simulink model "test storgrossenbeobachter"  (R2025b)
settings: Solver=ode23s  StartTime=0  StopTime=100  FixedStep=tStep  RelTol=1e-3  EnableMultiTasking=on
values from neighbouring files (symbols this model uses):
  A = [0 1 0 0 ... (first row only)    [test_init.m]    (also in zustandsregler.m)
  B = [0; -30.49; 0; 30.49]    [reglerInit.m]    (also in test_init.m; zustandsregler.m)
  C_new = [1 0 0 0 ... (first row only)    [reglerInit.m]    (also in test_init.m; zustandsregler.m)
  E_temp = zeros(4, 12)    [reglerInit.m]    (also in test_init.m)
  G = [1;1;1;1]    [reglerInit.m]    (also in test_init.m)
  Gamma_temp = zeros(6, 4)    [reglerInit.m]    (also in test_init.m)
  Kx = zeros(6, 4)    [reglerInit.m]    (also in test_init.m)
  Kxi = zeros(6,4)    [reglerInit.m]    (also in test_init.m)
  m1 = m1_sim    (= 1)    [test_init.m]    (also in zustandsregler.m)
  Pi_temp = zeros(4, 24)    [reglerInit.m]    (also in test_init.m)
  S_sy = [0 0 0 0 ... (first row only)    [reglerInit.m]    (also in test_init.m; zustandsregler.m)
  T = [0.3,1.2,1.5,1.7,1.7,3]    [reglerInit.m]    (also in test_init.m = [3,3,1.5,2,2.3,3]; zustandsregler.m = 50)
  x0 = [0; 0; 0; 0]    [reglerInit.m]    (also in test_init.m; zustandsregler.m = [0; 0; 1; 0])
  x_soll = 2    [test_init.m]
  xi0 = [0;0;0;0]    [reglerInit.m]    (also in test_init.m; zustandsregler.m = 0)
  zhut0 = [0;0;0;0]    [reglerInit.m]    (also in test_init.m; zustandsregler.m)
settings Model: Creator=Henning Schlüter  LastModifiedBy=marin
settings SolverCC: AlgebraicLoopSolver=TrustRegion
settings DataIOCC: SaveFormat=Array  SignalLoggingSaveFormat=ModelDataLogs  SaveOutput=off  SaveTime=off  ReturnWorkspaceOutputs=off
settings OptimizationCC: ExpressionDepthLimit=2147483647.0  LifeSpan=inf
settings DebuggingCC: UnderspecifiedInitializationDetection=Classic  MergeDetectMultiDrivingBlocksExec=none  SolverPrmCheckMsg=warning  UnconnectedInputMsg=warning  UnconnectedOutputMsg=warning  UnconnectedLineMsg=warning  StateNameClashWarn=warning  PregeneratedLibrarySubsystemCodeDiagnostic=none  SFUnexpectedBacktrackingDiag=warning  SFNoUnconditionalDefaultTransitionDiag=warning  SFExecutionAtInitializationDiag=none  ArithmeticOperatorsInVariantConditions=warning
settings HardwareCC: ProdBitPerPointer=32.0  ProdBitPerSizeT=32.0  ProdBitPerPtrDiffT=32.0  ProdLargestAtomicFloat=None  ProdIntDivRoundTo=Undefined  ProdEndianess=Unspecified  ProdWordSize=32.0  ProdHWDeviceType=32-bit Generic
settings ModelReferenceCC: EnableRefExpFcnMdlSchedulingChecks=on  PropagateSignalLabelsOutOfModel=off
settings SFSimCC: SimUseLocalCustomCode=off  CustomCodeUndefinedFunction=UseInterfaceOnly
settings RTWCC: RTWUseLocalCustomCode=off  GPUComputeCapability=3.5
settings CodeAppCC: StateflowObjectComments=on
settings GRTTargetCC: TargetLangStandard=C89/C90 (ANSI)  CombineOutputUpdateFcns=off  GRTInterface=on
settings ConfigComp: CovMetricSettings=dw  CovSaveCumulativeToWorkspaceVar=on  CovSaveSingleToWorkspaceVar=on  CovExternalEMLEnable=off  CovSFcnEnable=off

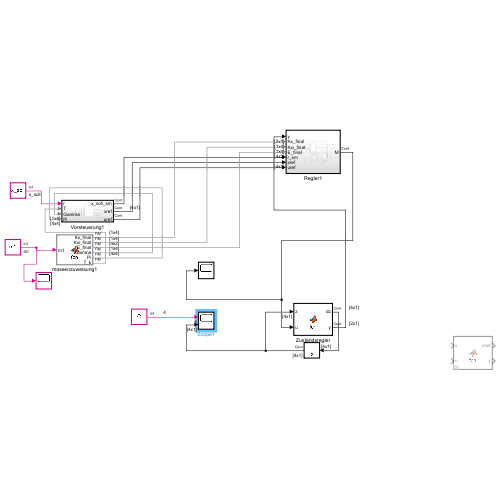
[thumbnail: Simulink's stored preview of the top-level diagram]
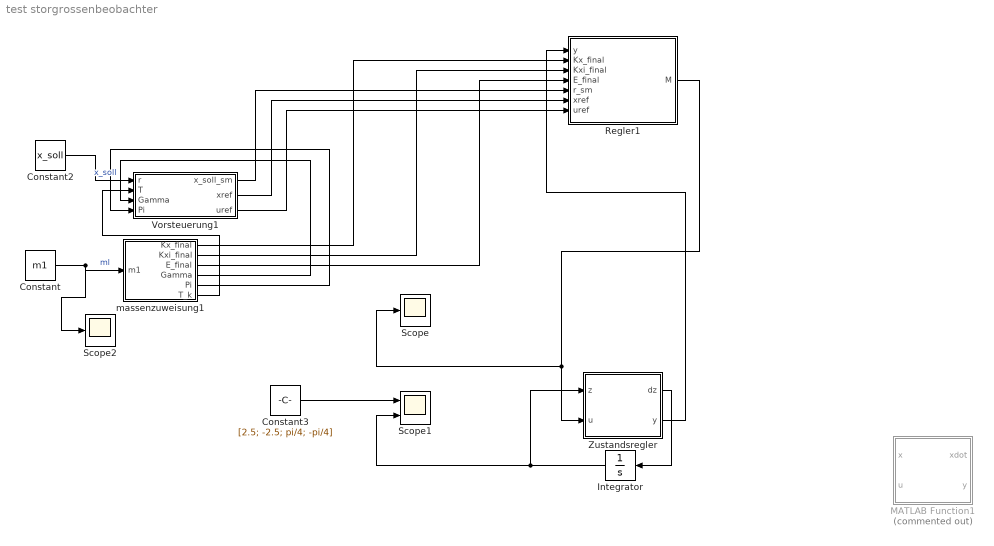
== system test storgrossenbeobachter ==
  Constant : Constant  Value=m1
  Constant2 : Constant  Value=x_soll
  Constant3 : Constant  Value=[2.5; -2.5; pi/4; -pi/4]
  Integrator : Integrator  InitialCondition=x0
  MATLAB Function1 : MATLAB Function  Commented=on  TreatAsAtomicUnit=on
  Regler1 : Subsystem
  Scope : Scope
      settings: ActiveDisplayYMinimum=-0.0045670835507599962  ActiveDisplayYMaximum=0.0070681602808915917  DataLoggingVariableName=ScopeData2
  Scope1 : Scope  NumInputPorts=2
      settings: MaximizeAxes=On  ActiveDisplayYMinimum=-1.292072495354522  ActiveDisplayYMaximum=1.1812647359995432  DataLoggingVariableName=ScopeData3
  Scope2 : Scope
      settings: ActiveDisplayYMinimum=-5.0106173887381429  ActiveDisplayYMaximum=5.5073930812373311  DataLoggingVariableName=ScopeData9
  Vorsteuerung1 : Subsystem
  Zustandsregler : MATLAB Function  TreatAsAtomicUnit=on
  massenzuweisung1 : MATLAB Function  TreatAsAtomicUnit=on
  wires:
  Regler1/1(M) -> Zustandsregler/2(u), Scope/1
  Vorsteuerung1/2(xref) -> Regler1/6(xref)
  Vorsteuerung1/1(x_soll_sm) -> Regler1/5(r_sm)
  massenzuweisung1/2(Kxi_final) -> Regler1/3(Kxi_final)
  Zustandsregler/2(y) -> Regler1/1(y)
  massenzuweisung1/3(E_final) -> Regler1/4(E_final)
  massenzuweisung1/6(T_k) -> Vorsteuerung1/2(T)
  massenzuweisung1/1(Kx_final) -> Regler1/2(Kx_final)
  Constant2/1 -> Vorsteuerung1/1(r)  "x_soll"
  Vorsteuerung1/3(uref) -> Regler1/7(uref)
  Zustandsregler/1(dz) -> Integrator/1
  Integrator/1 -> Zustandsregler/1(z), Scope1/2
  Constant/1 -> Scope2/1, massenzuweisung1/1(m1)  "ml"
  Constant3/1 -> Scope1/1
  massenzuweisung1/4(Gamma) -> Vorsteuerung1/3(Gamma)
  massenzuweisung1/5(Pi) -> Vorsteuerung1/4(Pi)

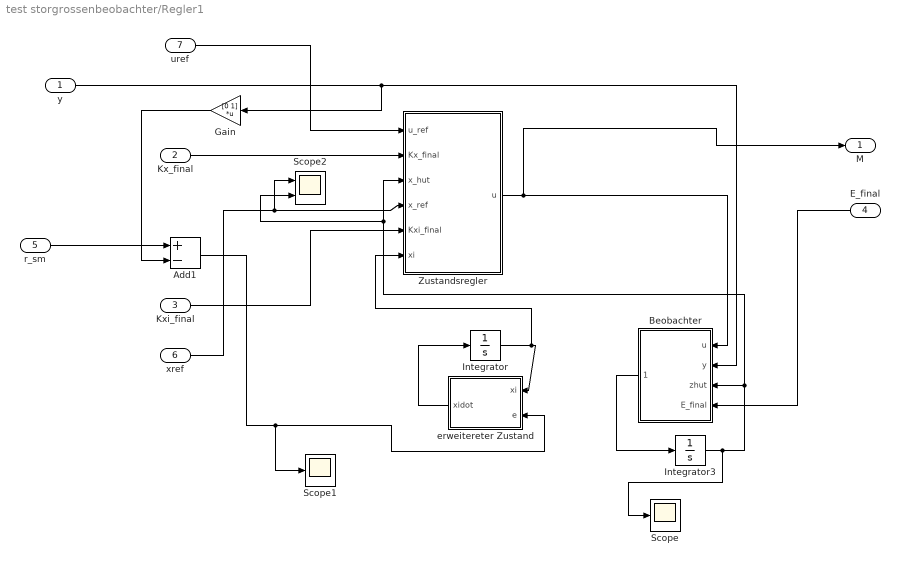
== system test storgrossenbeobachter/Regler1 ==
  y : Inport
  Kx_final : Inport  Port=2
  Kxi_final : Inport  Port=3
  E_final : Inport  Port=4
  r_sm : Inport  Port=5
  xref : Inport  Port=6
  uref : Inport  Port=7
  Add1 : Sum  Inputs=+-
  Beobachter : MATLAB Function  TreatAsAtomicUnit=on
  Gain : Gain  Gain=[0 1]  Multiplication=Matrix(K*u)
  Integrator : Integrator  InitialCondition=xi0
  Integrator3 : Integrator  InitialCondition=zhut0
  Scope : Scope
      settings: ActiveDisplayYMinimum=0.35119521026010936  ActiveDisplayYMaximum=0.989804365582628  DataLoggingVariableName=ScopeData6
  Scope1 : Scope
      settings: ActiveDisplayYMinimum=-0.10289845816979884  ActiveDisplayYMaximum=0.016663127287359483  DataLoggingVariableName=ScopeData7
  Scope2 : Scope  NumInputPorts=2
      settings: ActiveDisplayYMinimum=-0.13150511933969083  ActiveDisplayYMaximum=1.1257227910377408  DataLoggingVariableName=ScopeData8
  Zustandsregler : MATLAB Function  TreatAsAtomicUnit=on
  erweitereter Zustand : MATLAB Function  TreatAsAtomicUnit=on
  M : Outport
  wires:
  y/1 -> Beobachter/2(y), Gain/1
  Zustandsregler/1(u) -> Beobachter/1(u), M/1
  Gain/1 -> Add1/2
  r_sm/1 -> Add1/1
  uref/1 -> Zustandsregler/1(u_ref)
  xref/1 -> Scope2/1, Zustandsregler/4(x_ref)
  Kx_final/1 -> Zustandsregler/2(Kx_final)
  Kxi_final/1 -> Zustandsregler/5(Kxi_final)
  erweitereter Zustand/1(xidot) -> Integrator/1
  Integrator/1 -> Zustandsregler/6(xi), erweitereter Zustand/1(xi)
  Add1/1 -> Scope1/1, erweitereter Zustand/2(e)
  E_final/1 -> Beobachter/4(E_final)
  Beobachter/1(zhutdot) -> Integrator3/1
  Integrator3/1 -> Scope/1, Zustandsregler/3(x_hut), Scope2/2, Beobachter/3(zhut)

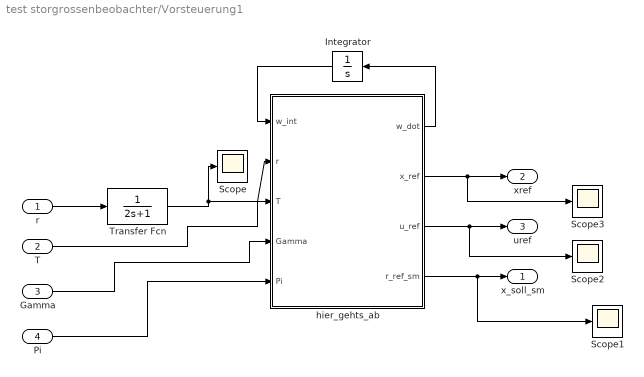
== system test storgrossenbeobachter/Vorsteuerung1 ==
  r : Inport
  T : Inport  Port=2
  Gamma : Inport  Port=3
  Pi : Inport  Port=4
  Integrator : Integrator  InitialCondition=[0;0;0]
  Scope{,1..3} (4 alike) : Scope
      Scope settings: ActiveDisplayYMinimum=-4.3163900712363112  ActiveDisplayYMaximum=0.46224694434276259  DataLoggingVariableName=ScopeData4
      Scope1 settings: ActiveDisplayYMinimum=-0.30966624511673135  ActiveDisplayYMaximum=1.9922091646276185  DataLoggingVariableName=ScopeData5
      Scope2 settings: ActiveDisplayYMinimum=-1.5301190889713152  ActiveDisplayYMaximum=1.2810123770175244
      Scope3 settings: ActiveDisplayYMinimum=-2.7580208827197352  ActiveDisplayYMaximum=0.32218794447761123
  Transfer Fcn : TransferFcn  Denominator=[2 1]
  hier_gehts_ab : MATLAB Function  TreatAsAtomicUnit=on
  x_soll_sm : Outport
  xref : Outport  Port=2
  uref : Outport  Port=3
  wires:
  hier_gehts_ab/1(w_dot) -> Integrator/1
  Integrator/1 -> hier_gehts_ab/1(w_int)
  r/1 -> Transfer Fcn/1
  hier_gehts_ab/2(x_ref) -> Scope3/1, xref/1
  hier_gehts_ab/3(u_ref) -> Scope2/1, uref/1
  hier_gehts_ab/4(r_ref_sm) -> Scope1/1, x_soll_sm/1
  T/1 -> hier_gehts_ab/3(T)
  Transfer Fcn/1 -> Scope/1, hier_gehts_ab/2(r)
  Gamma/1 -> hier_gehts_ab/4(Gamma)
  Pi/1 -> hier_gehts_ab/5(Pi)

== matlab function test storgrossenbeobachter/Regler1/erweitereter Zustand ==
  data: xi input; xidot output; e input; G parameter; S_sy parameter
function xidot = fcn(xi, e, G, S_sy)

Sxi = S_sy;

xidot = Sxi*xi+G*e;

== matlab function test storgrossenbeobachter/Vorsteuerung1/hier_gehts_ab ==
  data: w_int input; w_dot output; r input; Q_sy parameter; T input; x_ref output; u_ref output; r_ref_sm output; Gamma input; Pi input
function [w_dot, x_ref, u_ref, r_ref_sm] = fcn(w_int, r, Q_sy, T, Gamma, Pi)
    % 1. EXPLIZITE GRÖßENZUWEISUNG FÜR DIE AUSGÄNGE (Pre-Allocation)
    % Das bricht den Teufelskreis der Simulink-Größenerkennung am Integrator!
    w_dot = zeros(3, 1);
    x_ref = zeros(4, 1);

    % 2. Eingänge sicher machen
    r_val = double(r(1));                
    T_val = max(double(T(1)), 0.001);    
    w_vec = double(w_int(:));            % Zwingt w_int in einen [3x1] Spaltenvektor
    
    % 3. Workspace-Parameter sicher machen
    Pi_mat = double(Pi);                 
    Gam_vec = double(Gamma(:)');         
    Q_vec = double(Q_sy(:)');            

    % =========================================================
    % 4. Mathematik
    % =========================================================
    A_f = [0, 1, 0; 
           0, 0, 1; 
           -1/(T_val^3), -3/(T_val^2), -3/T_val];
           
    B_f = [0; 0; 1/(T_val^3)];
    
    % 5. Zuweisung in die fest reservierten Variablen
    % Das (:) verbietet Simulink jegliche eigenmächtige Größenänderung!
    w_dot(:) = A_f * w_vec + B_f * r_val;
    
    w = [r_val; w_vec];
    
    x_ref(:) = Pi_mat * w;
    u_ref = Gam_vec * w;
    r_ref_sm = Q_vec * w;
end

== matlab function test storgrossenbeobachter/Zustandsregler ==
  data: z input; dz output; u input; y output
function [dz, y] = fcn(z, u)
    
    % Parameter
    l = 1;
    m_1 = 1;
    m_s = 0.8;
    r = 0.041;
    g = 9.81;
    k_r = 7.2e-3;
    
    % Zustände extrahieren (zur besseren Lesbarkeit)
    z1 = z(1);
    z2 = z(2);
    z3 = z(3);
    z4 = z(4);
    
    % Nenner-Term
    N = -m_1*cos(z1)^2 + m_1 + m_s; 
    
    % Nichtlinearer Zustandsvektor dz/dt = f(z,u)
    dz = zeros(4,1); 
    
    dz(1) = z2;
    dz(2) = -(l*m_1*r*cos(z1)*sin(z1)*z2^2 + u*cos(z1) + g*m_1*r*sin(z1) + g*m_s*r*sin(z1) - k_r*r*z4*cos(z1)) / (l*r*N);
    dz(3) = z4;
    dz(4) =  (l*m_1*r*sin(z1)*z2^2 + u - k_r*r*z4 + g*m_1*r*cos(z1)*sin(z1)) / (r*N);
    

    y = [z1; z3];

== matlab function test storgrossenbeobachter/massenzuweisung1 ==
  data: m1 input; Kx parameter; Kxi parameter; E_temp parameter; Kx_final output; Kxi_final output; E_final output; Pi_temp parameter; Gamma_temp parameter; Gamma output; Pi output; T parameter; T_k output
function [Kx_final, Kxi_final, E_final, Gamma, Pi,T_k]= fcn(m1, Kx, Kxi, E_temp, Pi_temp, Gamma_temp, T)

E_final = zeros(4,2);
Kx_final = zeros(1,4);
Kxi_final = zeros(1,4);
Gamma = zeros(1,4);
Pi = zeros(4,4);
T_k = 0;

for i =1:6
    if (m1>i-1 && m1<=i)
        Kx_final = Kx(i,:);
        Kxi_final = Kxi(i,:);
        E_final = E_temp(:,2*i-1:2*i);
        Gamma = Gamma_temp(i, :);
        Pi = Pi_temp(:,4*i-3:4*i);
        T_k = T(i);
    
    end
end

== matlab function test storgrossenbeobachter/MATLAB Function1 ==
  data: x input; u input; xdot output; y output; B parameter; A parameter; C_new parameter
function [xdot,y] = fcn(x, u, B, A, C_new)

xdot= A*x+B*u;

y = C_new*x;

== matlab function test storgrossenbeobachter/Regler1/Beobachter ==
  data: u input; zhutdot output; y input; zhut input; A parameter; B parameter; C_new parameter; E_final input
function zhutdot = fcn(u, y, zhut, A, B, C_new, E_final)


zhutdot = (A-E_final*C_new)*zhut +B*u+E_final*y;

== matlab function test storgrossenbeobachter/Regler1/Zustandsregler ==
  data: u_ref input; u output; Kx_final input; x_hut input; x_ref input; Kxi_final input; xi input
function u = fcn(u_ref,Kx_final, x_hut, x_ref, Kxi_final,xi)

u = - Kx_final*(x_ref-x_hut)+Kxi_final*xi +  u_ref ;
